simulink model "gm_sampleModel1858_sub"  (R2023a)
settings: Solver=VariableStepAuto  StartTime=0.0  StopTime=10.0  RelTol=1e-3
libraries: hdlsllib x2, simulink x1
settings Model: Creator=user1  LastModifiedBy=user1
settings OptimizationCC: BlockReduction=off  ConditionallyExecuteInputs=off
settings DebuggingCC: InheritedTsInSrcMsg=none

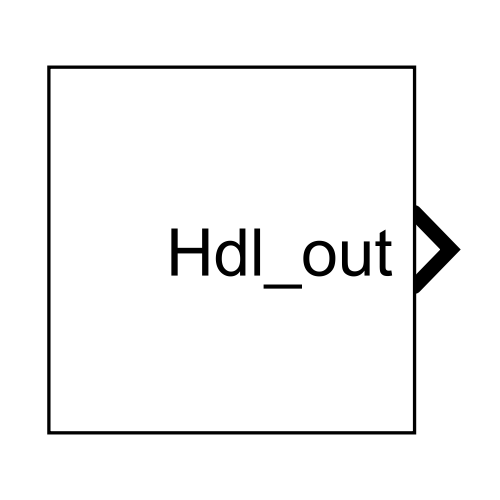
[thumbnail: Simulink's stored preview of the top-level diagram]
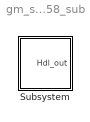
== system gm_sampleModel1858_sub ==
  Subsystem : Subsystem

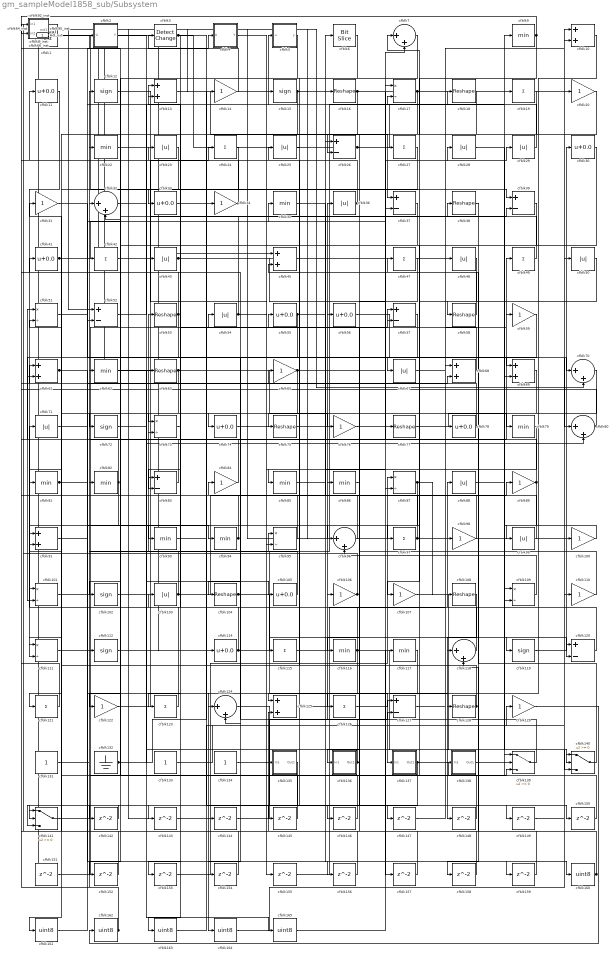
== system gm_sampleModel1858_sub/Subsystem ==
  cfblk1 : hdlsllib/Logic and Bit Operations/Interval Test  IntervalClosedRight=on  uplimit=0.5  IntervalClosedLeft=on  lowlimit=-0.5  OutDataTypeStr=uint8
  cfblk{10,13,45,61,68..69,91,125} (8 alike) : Sum  OutDataTypeStr=uint8
  cfblk{14,20,31,34,59,65,76,84,89,98,100,106..107,110,122,129} (16 alike) : Gain  OutDataTypeStr=uint8
  cfblk{17,51,73,87,95,101,109,111} (8 alike) : Product  Inputs=*/  OutDataTypeStr=uint8  RndMeth=Zero  SaturateOnIntegerOverflow=on
  cfblk{12,15,72,102,112,119} (6 alike) : Signum
  cfblk{23,25,28..29,36,43,48,50,54,67,71,88,99,103} (14 alike) : Abs  OutDataTypeStr=uint8  SaturateOnIntegerOverflow=off
  cfblk{16,18,38,53,58,63,75,77,104,108,128} (11 alike) : Reshape
  cfblk{11,30,33,41,55..56,74,78,105,114} (10 alike) : Bias  Bias=0.0  SaturateOnIntegerOverflow=off
  cfblk113_inst : Subsystem
  cfblk{19,24,27,42,47,49,97,115,121,123,126} (11 alike) : Sum  Inputs=+  OutDataTypeStr=uint8
  cfblk{9,22,35,62,79,81..82,85..86,93..94,116..117} (13 alike) : MinMax  OutDataTypeStr=uint8
  cfblk{7,32,70,80,96,118,124} (7 alike) : Sum  Inputs=|++  OutDataTypeStr=uint8
  cfblk{26,37,39,52,57,83,120,127} (8 alike) : Sum  Inputs=+-  OutDataTypeStr=uint8
  cfblk131 : Constant  OutDataTypeStr=uint8  SampleTime=-1
  cfblk132 : Ground
  cfblk133 : Constant  OutDataTypeStr=uint8  SampleTime=-1
  cfblk134 : Constant  OutDataTypeStr=uint8  SampleTime=-1
  cfblk135 : Subsystem
  cfblk136 : Subsystem
  cfblk137 : Subsystem
  cfblk138 : Subsystem
  cfblk139 : Switch  OutDataTypeStr=uint8  SaturateOnIntegerOverflow=off  InputSameDT=off
  cfblk140 : Switch  OutDataTypeStr=uint8  SaturateOnIntegerOverflow=off  InputSameDT=off
  cfblk141 : Switch  OutDataTypeStr=uint8  SaturateOnIntegerOverflow=off  InputSameDT=off
  cfblk{142..159} (18 alike) : Delay  SampleTime=1
  cfblk{160..165} (6 alike) : DataTypeConversion  OutDataTypeStr=uint8  SaturateOnIntegerOverflow=off  RndMeth=Floor
  cfblk2 : Subsystem  mask(Detect Fall Nonpositive){vinit=double(0), InputProcessing=Elements as channels (sample based), OutDataTypeStr=uint8}
      mask prompts: vinit "Simulink:masks:InitialCondition_MP"; InputProcessing "Simulink:masks:InputProcessing_MP"; OutDataTypeStr "Simulink:masks:OutputDataType_MP"
      mask help: Simulink:masks:DetectFallNonpositive_MD
      mask init:
      | InputProcessing = 'Elements as channels (sample based)';
      | OutDataTypeStr = 'uint8';
      | vinit = double(0);
      mask TypeOptions InputProcessing: Simulink:masks:ColumnsAsChannelsFrameBased | Simulink:masks:ElementsAsChannelsSampleBased
      mask TypeOptions OutDataTypeStr: Simulink:masks:uint8 | Simulink:masks:boolean
      mask Display: fprintf('U <= 0\n&  NOT\nU/z <= 0')
  cfblk21_inst : Subsystem
  cfblk3 : simulink/Logic and Bit Operations/Detect Change  vinit=0  OutDataTypeStr=uint8
      settings: LibrarySourceBlock=|
      | hdlsllib/Logic and Bit
      | Operations/Detect
      | Change
  cfblk4 : Subsystem  mask(Detect Rise Positive){vinit=double(0), InputProcessing=Elements as channels (sample based), OutDataTypeStr=uint8}
      mask prompts: vinit "Simulink:masks:InitialCondition_MP"; InputProcessing "Simulink:masks:InputProcessing_MP"; OutDataTypeStr "Simulink:masks:OutputDataType_MP"
      mask help: Simulink:masks:DetectRisePositive_MD
      mask init:
      | InputProcessing = 'Elements as channels (sample based)';
      | OutDataTypeStr = 'uint8';
      | vinit = double(0);
      mask TypeOptions InputProcessing: Simulink:masks:ColumnsAsChannelsFrameBased | Simulink:masks:ElementsAsChannelsSampleBased
      mask TypeOptions OutDataTypeStr: Simulink:masks:uint8 | Simulink:masks:boolean
      mask Display: fprintf('U > 0\n&  NOT\nU/z > 0')
  cfblk40_inst : Subsystem
  cfblk44_inst : Subsystem
  cfblk46_inst : Subsystem
  cfblk5 : Subsystem  mask(Compare To Constant){relop=<=, const=double(3), OutDataTypeStr=uint8, ZeroCross=on}
      mask prompts: relop "Simulink:masks:Operator_MP"; const "Simulink:masks:ConstantValue_MP"; OutDataTypeStr "Simulink:masks:OutputDataType_MP"; ZeroCross "Simulink:masks:EnableZerocrossingDetection_MP"
      mask help: Simulink:masks:CompareToConstant_MD
      mask init:
      | OutDataTypeStr = 'uint8';
      | ZeroCross = 'on';
      | blkName = 'sampleModel1858_sub/Subsystem/cfblk5';
      | const = double(3);
      | const_str = '3.0';
      | const_val = double(3);
      | relop = '<=';
      | setValue = 'fixdt(0, 8)';
      | str = '<= 3';
      mask TypeOptions relop: == | ~= | < | <= | >= | >
      mask TypeOptions OutDataTypeStr: Simulink:masks:uint8 | Simulink:masks:boolean
      mask Callback ZeroCross: sl('zeroCrossEnable', gcbh);
      mask Display: disp(str)
  cfblk6 : hdlsllib/Logic and Bit Operations/Bit Slice  lidx=7  ridx=0
  cfblk60_inst : Subsystem
  cfblk64_inst : Subsystem
  cfblk66_inst : Subsystem
  cfblk8_inst : Subsystem
  cfblk90_inst : Subsystem
  cfblk92_inst : Subsystem
  Hdl_out : Outport  OutDataTypeStr=uint8  SampleTime=1
  wires:
  cfblk1/1 -> cfblk39/1
  cfblk10/1 -> cfblk125/1
  cfblk100/1 -> cfblk99/1
  cfblk101/1 -> cfblk95/1
  cfblk102/1 -> cfblk24/1
  cfblk103/1 -> cfblk53/1, cfblk89/1, cfblk73/2
  cfblk104/1 -> cfblk120/2, cfblk137/1(In1)
  cfblk105/1 -> cfblk12/1
  cfblk106/1 -> cfblk66_inst/1(in1), cfblk22/1
  cfblk107/1 -> cfblk140/2
  cfblk108/1 -> cfblk148/1
  cfblk109/1 -> cfblk96/2
  cfblk11/1 -> cfblk111/2
  cfblk110/1 -> cfblk84/1
  cfblk111/1 -> cfblk57/1
  cfblk112/1 -> cfblk114/1
  cfblk113_inst/1(out1) -> cfblk20/1
  cfblk114/1 -> cfblk18/1, cfblk13/1
  cfblk115/1 -> cfblk119/1
  cfblk116/1 -> cfblk54/1, cfblk140/3, cfblk128/1, cfblk124/2
  cfblk117/1 -> cfblk164/1
  cfblk118/1 -> cfblk32/2
  cfblk119/1 -> cfblk30/1
  cfblk12/1 -> cfblk155/1
  cfblk120/1 -> cfblk88/1
  cfblk121/1 -> cfblk90_inst/1(in1)
  cfblk122/1 -> cfblk49/1
  cfblk123/1 -> cfblk71/1
  cfblk124/1 -> cfblk149/1
  cfblk125/1 -> cfblk36/1
  cfblk126/1 -> cfblk127/1
  cfblk127/1 -> cfblk29/1
  cfblk128/1 -> cfblk91/2, cfblk55/1
  cfblk129/1 -> cfblk162/1
  cfblk13/1 -> cfblk37/1
  cfblk131/1 -> cfblk62/1
  cfblk132/1 -> cfblk63/1, cfblk34/1
  cfblk133/1 -> cfblk110/1
  cfblk134/1 -> cfblk106/1
  cfblk135/1(Out1) -> cfblk141/2
  cfblk136/1(Out1) -> cfblk103/1, cfblk86/1
  cfblk137/1(Out1) -> cfblk141/3, cfblk139/3, cfblk17/2
  cfblk138/1(Out1) -> cfblk19/1
  cfblk139/1 -> cfblk41/1
  cfblk14/1 -> cfblk3/1
  cfblk140/1 -> cfblk47/1
  cfblk141/1 -> cfblk139/2
  cfblk142/1 -> cfblk141/1
  cfblk143/1 -> cfblk139/1
  cfblk144/1 -> cfblk127/2
  cfblk145/1 -> cfblk61/1
  cfblk146/1 -> cfblk32/1
  cfblk147/1 -> cfblk39/2
  cfblk148/1 -> cfblk7/1
  cfblk149/1 -> cfblk10/2
  cfblk15/1 -> cfblk72/1, cfblk121/1
  cfblk150/1 -> cfblk101/1
  cfblk151/1 -> cfblk37/2
  cfblk152/1 -> cfblk64_inst/1(in1)
  cfblk153/1 -> cfblk87/1
  cfblk154/1 -> cfblk90_inst/2(in2)
  cfblk155/1 -> cfblk68/1
  cfblk156/1 -> cfblk51/2
  cfblk157/1 -> cfblk46_inst/2(in2)
  cfblk158/1 -> cfblk125/2
  cfblk159/1 -> cfblk118/2
  cfblk16/1 -> cfblk120/1, cfblk93/1
  cfblk160/1 -> cfblk66_inst/2(in2), cfblk56/1
  cfblk161/1 -> cfblk4/1(U)
  cfblk162/1 -> cfblk44_inst/1(in1), cfblk82/1
  cfblk163/1 -> cfblk129/1
  cfblk164/1 -> cfblk50/1
  cfblk165/1 -> cfblk117/1
  cfblk17/1 -> cfblk26/2, cfblk152/1
  cfblk18/1 -> cfblk85/1
  cfblk19/1 -> cfblk136/1(In1)
  cfblk2/1(Y) -> cfblk165/1
  cfblk20/1 -> cfblk146/1
  cfblk21_inst/1(out1) -> cfblk144/1
  cfblk22/1 -> cfblk135/1(In1)
  cfblk23/1 -> cfblk33/1
  cfblk24/1 -> cfblk161/1
  cfblk25/1 -> cfblk145/1
  cfblk26/1 -> Hdl_out/1, cfblk9/1
  cfblk27/1 -> cfblk153/1
  cfblk28/1 -> cfblk140/1
  cfblk29/1 -> cfblk5/1(u)
  cfblk3/1 -> cfblk83/2, cfblk147/1
  cfblk30/1 -> cfblk107/1
  cfblk31/1 -> cfblk69/1
  cfblk32/1 -> cfblk138/1(In1)
  cfblk33/1 -> cfblk67/1
  cfblk34/1 -> cfblk92_inst/1(in1), cfblk11/1
  cfblk35/1 -> cfblk87/2
  cfblk36/1 -> cfblk64_inst/2(in2), cfblk40_inst/2(in2)
  cfblk37/1 -> cfblk102/1
  cfblk38/1 -> cfblk158/1
  cfblk39/1 -> cfblk126/1
  cfblk4/1(Y) -> cfblk160/1
  cfblk40_inst/1(out1) -> cfblk16/1
  cfblk41/1 -> cfblk7/2, cfblk6/1
  cfblk42/1 -> cfblk14/1
  cfblk43/1 -> cfblk157/1, cfblk123/1
  cfblk44_inst/1(out1) -> cfblk52/1, cfblk151/1, cfblk115/1
  cfblk45/1 -> cfblk28/1
  cfblk46_inst/1(out1) -> cfblk48/1
  cfblk47/1 -> cfblk96/1
  cfblk48/1 -> cfblk97/1
  cfblk49/1 -> cfblk60_inst/1(in1)
  cfblk5/1(y) -> cfblk163/1
  cfblk50/1 -> cfblk58/1
  cfblk51/1 -> cfblk35/1
  cfblk52/1 -> cfblk15/1
  cfblk53/1 -> cfblk61/2, cfblk21_inst/1(in1)
  cfblk54/1 -> cfblk92_inst/2(in2), cfblk70/1
  cfblk55/1 -> cfblk83/1, cfblk69/2
  cfblk56/1 -> cfblk80/1
  cfblk57/1 -> cfblk101/2
  cfblk58/1 -> cfblk25/1
  cfblk59/1 -> cfblk104/1
  cfblk6/1 -> cfblk142/1
  cfblk60_inst/1(out1) -> cfblk70/2
  cfblk61/1 -> cfblk68/2, cfblk94/1
  cfblk62/1 -> cfblk80/2
  cfblk63/1 -> cfblk76/1, cfblk73/1, cfblk1/1
  cfblk64_inst/1(out1) -> cfblk45/1, cfblk98/1
  cfblk65/1 -> cfblk17/1, cfblk154/1
  cfblk66_inst/1(out1) -> cfblk43/1
  cfblk67/1 -> cfblk10/1
  cfblk68/1 -> cfblk23/1
  cfblk69/1 -> cfblk122/1
  cfblk7/1 -> cfblk75/1
  cfblk70/1 -> cfblk81/1
  cfblk71/1 -> cfblk156/1
  cfblk72/1 -> cfblk105/1
  cfblk73/1 -> cfblk143/1
  cfblk74/1 -> cfblk150/1
  cfblk75/1 -> cfblk118/1
  cfblk76/1 -> cfblk77/1
  cfblk77/1 -> cfblk79/1
  cfblk78/1 -> cfblk60_inst/2(in2), cfblk45/2
  cfblk79/1 -> cfblk95/2
  cfblk8_inst/1(out1) -> cfblk78/1
  cfblk80/1 -> cfblk74/1, cfblk44_inst/2(in2)
  cfblk81/1 -> cfblk52/2, cfblk13/2, cfblk124/1
  cfblk82/1 -> cfblk91/1, cfblk46_inst/1(in1)
  cfblk83/1 -> cfblk51/1
  cfblk84/1 -> cfblk31/1
  cfblk85/1 -> cfblk159/1
  cfblk86/1 -> cfblk116/1
  cfblk87/1 -> cfblk57/2, cfblk108/1, cfblk111/1
  cfblk88/1 -> cfblk109/1
  cfblk89/1 -> cfblk21_inst/2(in2), cfblk109/2
  cfblk9/1 -> cfblk113_inst/2(in2), cfblk27/1
  cfblk90_inst/1(out1) -> cfblk100/1
  cfblk91/1 -> cfblk112/1
  cfblk92_inst/1(out1) -> cfblk40_inst/1(in1)
  cfblk93/1 -> cfblk38/1
  cfblk94/1 -> cfblk113_inst/1(in1), cfblk2/1(U)
  cfblk95/1 -> cfblk8_inst/1(in1)
  cfblk96/1 -> cfblk26/1
  cfblk97/1 -> cfblk8_inst/2(in2), cfblk59/1
  cfblk98/1 -> cfblk42/1
  cfblk99/1 -> cfblk65/1

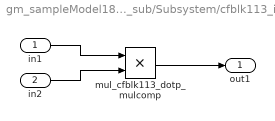
== system gm_sampleModel1858_sub/Subsystem/cfblk113_inst ==
  in1 : Inport  OutDataTypeStr=uint8  SampleTime=1
  in2 : Inport  Port=2  OutDataTypeStr=uint8  SampleTime=1
  mul_cfblk113_dotp_mulcomp : Product  Inputs=**  OutDataTypeStr=uint8  SampleTime=1
  out1 : Outport  OutDataTypeStr=uint8  SampleTime=1
  wires:
  in1/1 -> mul_cfblk113_dotp_mulcomp/1
  in2/1 -> mul_cfblk113_dotp_mulcomp/2
  mul_cfblk113_dotp_mulcomp/1 -> out1/1

== system gm_sampleModel1858_sub/Subsystem/cfblk135 ==
  In1 : Inport  OutDataTypeStr=uint8  PortDimensions=1  SampleTime=1
  Out1 : Outport  SampleTime=1
  wires:
  In1/1 -> Out1/1

== system gm_sampleModel1858_sub/Subsystem/cfblk136 ==
  In1 : Inport  OutDataTypeStr=uint8  PortDimensions=1  SampleTime=1
  Out1 : Outport  SampleTime=1
  wires:
  In1/1 -> Out1/1

== system gm_sampleModel1858_sub/Subsystem/cfblk137 ==
  In1 : Inport  OutDataTypeStr=uint8  PortDimensions=1  SampleTime=1
  Out1 : Outport  SampleTime=1
  wires:
  In1/1 -> Out1/1

== system gm_sampleModel1858_sub/Subsystem/cfblk138 ==
  In1 : Inport  OutDataTypeStr=uint8  PortDimensions=1  SampleTime=1
  Out1 : Outport  SampleTime=1
  wires:
  In1/1 -> Out1/1

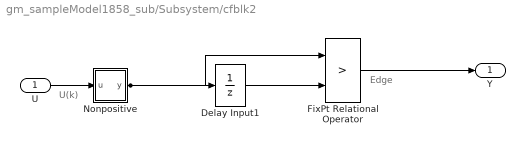
== system gm_sampleModel1858_sub/Subsystem/cfblk2 ==
  note: U(k)
  note: Edge
  U : Inport  OutDataTypeStr=uint8  SampleTime=1
  Delay Input1 : UnitDelay  Description=Store in Global RAM  DisableCoverage=on  InitialCondition=vinit  SampleTime=-1  HasFrameUpgradeWarning=on
  FixPt Relational Operator : RelationalOperator  Operator=>  OutDataTypeStr=fixdt(0, 8)  ZeroCross=off  InputSameDT=off
  Nonpositive : Subsystem  mask(Compare To Zero){relop=<=, OutDataTypeStr=boolean, ZeroCross=off}
      mask prompts: relop "Simulink:masks:Operator_MP"; OutDataTypeStr "Simulink:masks:OutputDataType_MP"; ZeroCross "Simulink:masks:EnableZerocrossingDetection_MP"
      mask help: Simulink:masks:CompareToZero_MD
      mask init:
      | OutDataTypeStr = 'boolean';
      | ZeroCross = 'off';
      | blkName = 'sampleModel1858_sub/Subsystem/cfblk2/Nonpositive';
      | relop = '<=';
      | setValue = 'boolean';
      mask TypeOptions relop: == | ~= | < | <= | >= | >
      mask TypeOptions OutDataTypeStr: Simulink:masks:uint8 | Simulink:masks:boolean
      mask Callback ZeroCross: sl('zeroCrossEnable', gcbh);
      mask Display: disp([relop,' 0'])
  Y : Outport  SampleTime=1
  wires:
  U/1 -> Nonpositive/1(u)
  Delay Input1/1 -> FixPt Relational Operator/2
  FixPt Relational Operator/1 -> Y/1
  Nonpositive/1(y) -> FixPt Relational Operator/1, Delay Input1/1

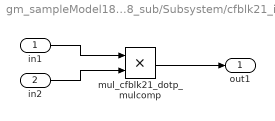
== system gm_sampleModel1858_sub/Subsystem/cfblk21_inst ==
  in1 : Inport  OutDataTypeStr=uint8  SampleTime=1
  in2 : Inport  Port=2  OutDataTypeStr=uint8  SampleTime=1
  mul_cfblk21_dotp_mulcomp : Product  Inputs=**  OutDataTypeStr=uint8  SampleTime=1
  out1 : Outport  OutDataTypeStr=uint8  SampleTime=1
  wires:
  in1/1 -> mul_cfblk21_dotp_mulcomp/1
  in2/1 -> mul_cfblk21_dotp_mulcomp/2
  mul_cfblk21_dotp_mulcomp/1 -> out1/1

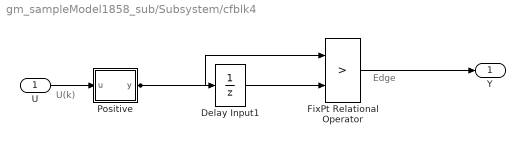
== system gm_sampleModel1858_sub/Subsystem/cfblk4 ==
  note: U(k)
  note: Edge
  U : Inport  OutDataTypeStr=uint8  SampleTime=1
  Delay Input1 : UnitDelay  Description=Store in Global RAM  DisableCoverage=on  InitialCondition=vinit  SampleTime=-1  HasFrameUpgradeWarning=on
  FixPt Relational Operator : RelationalOperator  Operator=>  OutDataTypeStr=fixdt(0, 8)  ZeroCross=off  InputSameDT=off
  Positive : Subsystem  mask(Compare To Zero){relop=>, OutDataTypeStr=boolean, ZeroCross=off}
      mask prompts: relop "Simulink:masks:Operator_MP"; OutDataTypeStr "Simulink:masks:OutputDataType_MP"; ZeroCross "Simulink:masks:EnableZerocrossingDetection_MP"
      mask help: Simulink:masks:CompareToZero_MD
      mask init:
      | OutDataTypeStr = 'boolean';
      | ZeroCross = 'off';
      | blkName = 'sampleModel1858_sub/Subsystem/cfblk4/Positive';
      | relop = '>';
      | setValue = 'boolean';
      mask TypeOptions relop: == | ~= | < | <= | >= | >
      mask TypeOptions OutDataTypeStr: Simulink:masks:uint8 | Simulink:masks:boolean
      mask Callback ZeroCross: sl('zeroCrossEnable', gcbh);
      mask Display: disp([relop,' 0'])
  Y : Outport  SampleTime=1
  wires:
  U/1 -> Positive/1(u)
  Delay Input1/1 -> FixPt Relational Operator/2
  FixPt Relational Operator/1 -> Y/1
  Positive/1(y) -> FixPt Relational Operator/1, Delay Input1/1

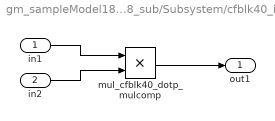
== system gm_sampleModel1858_sub/Subsystem/cfblk40_inst ==
  in1 : Inport  OutDataTypeStr=uint8  SampleTime=1
  in2 : Inport  Port=2  OutDataTypeStr=uint8  SampleTime=1
  mul_cfblk40_dotp_mulcomp : Product  Inputs=**  OutDataTypeStr=uint8  SampleTime=1
  out1 : Outport  OutDataTypeStr=uint8  SampleTime=1
  wires:
  in1/1 -> mul_cfblk40_dotp_mulcomp/1
  in2/1 -> mul_cfblk40_dotp_mulcomp/2
  mul_cfblk40_dotp_mulcomp/1 -> out1/1

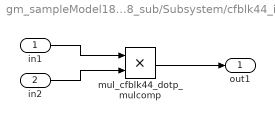
== system gm_sampleModel1858_sub/Subsystem/cfblk44_inst ==
  in1 : Inport  OutDataTypeStr=uint8  SampleTime=1
  in2 : Inport  Port=2  OutDataTypeStr=uint8  SampleTime=1
  mul_cfblk44_dotp_mulcomp : Product  Inputs=**  OutDataTypeStr=uint8  SampleTime=1
  out1 : Outport  OutDataTypeStr=uint8  SampleTime=1
  wires:
  in1/1 -> mul_cfblk44_dotp_mulcomp/1
  in2/1 -> mul_cfblk44_dotp_mulcomp/2
  mul_cfblk44_dotp_mulcomp/1 -> out1/1

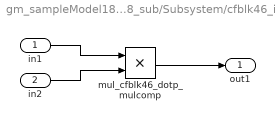
== system gm_sampleModel1858_sub/Subsystem/cfblk46_inst ==
  in1 : Inport  OutDataTypeStr=uint8  SampleTime=1
  in2 : Inport  Port=2  OutDataTypeStr=uint8  SampleTime=1
  mul_cfblk46_dotp_mulcomp : Product  Inputs=**  OutDataTypeStr=uint8  SampleTime=1
  out1 : Outport  OutDataTypeStr=uint8  SampleTime=1
  wires:
  in1/1 -> mul_cfblk46_dotp_mulcomp/1
  in2/1 -> mul_cfblk46_dotp_mulcomp/2
  mul_cfblk46_dotp_mulcomp/1 -> out1/1

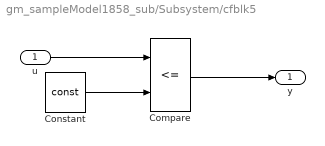
== system gm_sampleModel1858_sub/Subsystem/cfblk5 ==
  u : Inport  OutDataTypeStr=uint8  SampleTime=1
  Compare : RelationalOperator  Operator=<=  OutDataTypeStr=fixdt(0, 8)
  Constant : Constant  DisableCoverage=on  Value=const  OutDataTypeStr=Inherit: Inherit via back propagation  SampleTime=-1
  y : Outport  SampleTime=1
  wires:
  u/1 -> Compare/1
  Compare/1 -> y/1
  Constant/1 -> Compare/2

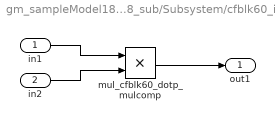
== system gm_sampleModel1858_sub/Subsystem/cfblk60_inst ==
  in1 : Inport  OutDataTypeStr=uint8  SampleTime=1
  in2 : Inport  Port=2  OutDataTypeStr=uint8  SampleTime=1
  mul_cfblk60_dotp_mulcomp : Product  Inputs=**  OutDataTypeStr=uint8  SampleTime=1
  out1 : Outport  OutDataTypeStr=uint8  SampleTime=1
  wires:
  in1/1 -> mul_cfblk60_dotp_mulcomp/1
  in2/1 -> mul_cfblk60_dotp_mulcomp/2
  mul_cfblk60_dotp_mulcomp/1 -> out1/1

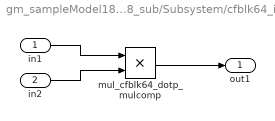
== system gm_sampleModel1858_sub/Subsystem/cfblk64_inst ==
  in1 : Inport  OutDataTypeStr=uint8  SampleTime=1
  in2 : Inport  Port=2  OutDataTypeStr=uint8  SampleTime=1
  mul_cfblk64_dotp_mulcomp : Product  Inputs=**  OutDataTypeStr=uint8  SampleTime=1
  out1 : Outport  OutDataTypeStr=uint8  SampleTime=1
  wires:
  in1/1 -> mul_cfblk64_dotp_mulcomp/1
  in2/1 -> mul_cfblk64_dotp_mulcomp/2
  mul_cfblk64_dotp_mulcomp/1 -> out1/1

== system gm_sampleModel1858_sub/Subsystem/cfblk66_inst ==
  in1 : Inport  OutDataTypeStr=uint8  SampleTime=1
  in2 : Inport  Port=2  OutDataTypeStr=uint8  SampleTime=1
  mul_cfblk66_dotp_mulcomp : Product  Inputs=**  OutDataTypeStr=uint8  SampleTime=1
  out1 : Outport  OutDataTypeStr=uint8  SampleTime=1
  wires:
  in1/1 -> mul_cfblk66_dotp_mulcomp/1
  in2/1 -> mul_cfblk66_dotp_mulcomp/2
  mul_cfblk66_dotp_mulcomp/1 -> out1/1

== system gm_sampleModel1858_sub/Subsystem/cfblk8_inst ==
  in1 : Inport  OutDataTypeStr=uint8  SampleTime=1
  in2 : Inport  Port=2  OutDataTypeStr=uint8  SampleTime=1
  mul_cfblk8_dotp_mulcomp : Product  Inputs=**  OutDataTypeStr=uint8  SampleTime=1
  out1 : Outport  OutDataTypeStr=uint8  SampleTime=1
  wires:
  in1/1 -> mul_cfblk8_dotp_mulcomp/1
  in2/1 -> mul_cfblk8_dotp_mulcomp/2
  mul_cfblk8_dotp_mulcomp/1 -> out1/1

== system gm_sampleModel1858_sub/Subsystem/cfblk90_inst ==
  in1 : Inport  OutDataTypeStr=uint8  SampleTime=1
  in2 : Inport  Port=2  OutDataTypeStr=uint8  SampleTime=1
  mul_cfblk90_dotp_mulcomp : Product  Inputs=**  OutDataTypeStr=uint8  SampleTime=1
  out1 : Outport  OutDataTypeStr=uint8  SampleTime=1
  wires:
  in1/1 -> mul_cfblk90_dotp_mulcomp/1
  in2/1 -> mul_cfblk90_dotp_mulcomp/2
  mul_cfblk90_dotp_mulcomp/1 -> out1/1

== system gm_sampleModel1858_sub/Subsystem/cfblk92_inst ==
  in1 : Inport  OutDataTypeStr=uint8  SampleTime=1
  in2 : Inport  Port=2  OutDataTypeStr=uint8  SampleTime=1
  mul_cfblk92_dotp_mulcomp : Product  Inputs=**  OutDataTypeStr=uint8  SampleTime=1
  out1 : Outport  OutDataTypeStr=uint8  SampleTime=1
  wires:
  in1/1 -> mul_cfblk92_dotp_mulcomp/1
  in2/1 -> mul_cfblk92_dotp_mulcomp/2
  mul_cfblk92_dotp_mulcomp/1 -> out1/1

== system gm_sampleModel1858_sub/Subsystem/cfblk2/Nonpositive ==
  u : Inport  OutDataTypeStr=uint8  SampleTime=1
  Compare : RelationalOperator  Operator=<=  OutDataTypeStr=boolean  ZeroCross=off
  Constant : Constant  DisableCoverage=on  Value=0  OutDataTypeStr=Inherit: Inherit via back propagation  SampleTime=-1  PreserveConstantTs=on
  y : Outport  SampleTime=1
  wires:
  u/1 -> Compare/1
  Compare/1 -> y/1
  Constant/1 -> Compare/2

== system gm_sampleModel1858_sub/Subsystem/cfblk4/Positive ==
  u : Inport  OutDataTypeStr=uint8  SampleTime=1
  Compare : RelationalOperator  Operator=>  OutDataTypeStr=boolean  ZeroCross=off
  Constant : Constant  DisableCoverage=on  Value=0  OutDataTypeStr=Inherit: Inherit via back propagation  SampleTime=-1  PreserveConstantTs=on
  y : Outport  SampleTime=1
  wires:
  u/1 -> Compare/1
  Compare/1 -> y/1
  Constant/1 -> Compare/2
